simulink model "sim1"  (R2013a)
settings: Solver=ode45  StartTime=0.0  StopTime=10.0  RelTol=1e-3
libraries: simulink x1
settings Model: Creator=Pires  LastModifiedBy=Pires

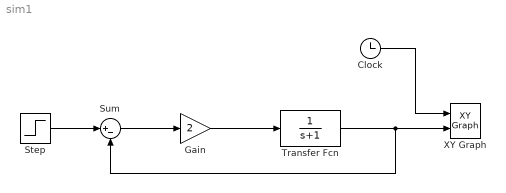
== system sim1 ==
  Clock : Clock
  Gain : Gain  Gain=2
  Step : Step  SampleTime=0
  Sum : Sum  Inputs=|+-
  Transfer Fcn : TransferFcn  Denominator=[1 1]
  XY Graph : simulink/Sinks/XY Graph  xmin=0  xmax=10  ymin=0  ymax=1  st=-1
  wires:
  Step/1 -> Sum/1
  Gain/1 -> Transfer Fcn/1
  Sum/1 -> Gain/1
  Transfer Fcn/1 -> XY Graph/2, Sum/2
  Clock/1 -> XY Graph/1
